simulink library "EngineSystemSubmodel"  (Simulink 8.1)
settings: Solver=ode45  StartTime=0.0  StopTime=10.0  FixedStep=1e-4  RelTol=1e-3
values from neighbouring files (symbols this model uses):
  B = [B1;B2]    [GensetRespOptimiztion.m]    (also in GensetRespOptimiztionTorstein.m; Init8RTFLEX68D.m = 0.68; init_MVM.m = 0.127)
  beta = 0.75    [Init8RTFLEX68D.m]
  cAStartRef = 104.8    [Init8RTFLEX68D.m]
  coeffMechEff = [0.135;0.155]    [Init8RTFLEX68D.m]
  comp_eff_map = [0 0 0 0 0 0 0 0 0 0 0 0 ... (250000 elements, 500x500)]    [comp_map.mat]    (also in comp_mapABB A175-35L.mat)
  comp_flow_map = [0 0 0 0 0 0 0 0 0 0 0 0 ... (250000 elements, 500x500)]    [comp_map.mat]    (also in comp_mapABB A175-35L.mat)
  D_turb_wheel = TC.TC_map.turb.D_wheel    [init_MVM.m]
  dCALiftDown = cAVVDownRef(end) - cAVVDownRef(1)    [Init8RTFLEX68D.m]
  dCALiftTopRef = 63.5    [Init8RTFLEX68D.m]
  dCALiftUp = cAVVUpRef(end) - cAVVUpRef(1)    [Init8RTFLEX68D.m]
  Dp = 0.383    [Init8RTFLEX68D.m]
  Ds = 0.079    [Init8RTFLEX68D.m]
  Dv = 0.425    [Init8RTFLEX68D.m]
  eff_coeff = [-1.0889528323728;0.91854258409396;-0.10659748546926;                     0.21229452390244;-0.053186221596493;-0.005451194709834]    [Init8RTFLEX68D.m]
  eta_turb_max = TC.TC_map.turb.eff_max    [init_MVM.m]
  flow_coeff_turb = [-1.585326540339;-4.823836967181;1.5853156139822]    [Init8RTFLEX68D.m]    (also in init_MVM.m = TC.TC_map.turb.flow_fit_coeff)
  fs = 0.0683    [Init8RTFLEX68D.m]    (also in NOxProcessGUI.m = varargin{2}; initHybrid.m; initMV.m; init_MVM.m = 0.0682925799315)
  genset = generators(1)    [runTempCyl4S.m]
  J_tc = TC.SAE_map_comp.inertia    [init_MVM.m]
  jShaft = 0    [EngineSystemParameters.m]    (also in Init8RTFLEX68D.m = 323000)
  jTC = 2    [Init8RTFLEX68D.m]
  Kb = 1*ones(engines,1)    [initHybrid.m]    (also in initMV.m; init_MVM.m = 1; init_ele.m = 1)
  Kd = 20*ones(engines,1)    [initHybrid.m]    (also in initMV.m; init_MVM.m = 10; init_ele.m = 20)
  Ki = 20*ones(engines,1)    [initHybrid.m]    (also in initMV.m; init_MVM.m = 10; init_ele.m = 20)
  Kp = 20*ones(engines,1)    [initHybrid.m]    (also in initMV.m; init_MVM.m = 10; init_ele.m = 20)
  lambdaCrank = 0.5056    [Init8RTFLEX68D.m]
  liftMax = 0.17    [Init8RTFLEX68D.m]
  Load_amp = x(4) + xRef(i)    [GetErrGensetResp.m]    (also in runsimulation.m = 0.55; runsimulationRecovery.m = InitialLoad(jj) + LoadStep(ii))
  Load_bias = x(4)    [GetErrGensetResp.m]    (also in runsimulation.m = 0.15; runsimulationRecovery.m = InitialLoad(jj))
  Load_index = 1    [GetErrGensetResp.m]    (also in runsimulation.m; runsimulationRecovery.m)
  mqfCycMax = 9.5547e-2    (= 0.095547)    [Init8RTFLEX68D.m]
  N = x*noMol    [NOxProcessGUI.m]    (also in initHybrid.m = .1*ones(engines,1); initMV.m = .1*ones(engines,1); init_ele.m = 0.1)
  n288_rep = [0 222.054 444.108 666.162 888.216 1110.27 1332.324 1554.378 1776.432 1998.486 2220.54 2442.594 ... (500 elements, 1x500)]    [comp_map.mat]
  nPort = 28    [Init8RTFLEX68D.m]
  npr = length(pr_rep)    [Init8RTFLEX68D.m]    (also in initHybrid.m; initMV.m; init_MVM.m)
  nsp = length(n288_rep)    [Init8RTFLEX68D.m]    (also in initHybrid.m; initMV.m; init_MVM.m)
  nStroke = 2    [Init8RTFLEX68D.m]
  omegat0 = RPM_TC_initial/30*pi    [init_MVM.m]
  pr_rep = [1.01 1.0150249672 1.0200499344 1.0250749016 1.0300998688 1.035124836 1.0401498032 1.0451747704 1.0501997376 1.0552247048 1.060249672 1.0652746392 ... (500 elements, 1x500)]    [comp_map.mat]
  r = 0.035    [Init8RTFLEX68D.m]
  Start_time = 50    [GetErrGensetResp.m]    (also in runsimulation.m; runsimulationRecovery.m)
  stroke = 2.72    [Init8RTFLEX68D.m]
  T_load = 1    [GetErrGensetResp.m]    (also in runsimulation.m; runsimulationRecovery.m)
  T_ref_turb = TC.TC_map.turb.T_ref    [init_MVM.m]
  u0 = 0.2    [init_MVM.m]
  Uc_opt = TC.TC_map.turb.Uc_opt    [init_MVM.m]
  w = 0.021    [Init8RTFLEX68D.m]
  wasteGateMax = 10    [Init8RTFLEX68D.m]
  wasteGateMin = 0    [Init8RTFLEX68D.m]
  wiebePara = [0.07;0.57;3.05;11;24;56.3;1.5;1;0.7]    [Init8RTFLEX68D.m]
  X = 0.07    [Init8RTFLEX68D.m]
  Y = 0.16    [Init8RTFLEX68D.m]
undefined symbols (not defined in the file or in its folder): aCrank, cAVVDownRef, cAVVUpRef, liftDownRef, liftUpRef, omega0, Td, Ti, u_max
undefined symbols (not defined in the file): BWdmExhBypass, cAlpha, cCylHT, E0A, ECyl0, hn, KbWG, KpWG, lowerCloseSPWG, m0A, mb0A, mbCyl0, mCp, mCyl0, nCyl, phi0, phi0A, phi0rad, RPM0, RPMMax, RPMT0, TiWG, upperOpenWG, V0A, vCyl0, wasteGateRatio
libraries: EngineSystemSubmodel x49, simulink x1
(part 1 of 3)
settings Model: Creator=yum  LastModifiedBy=yum

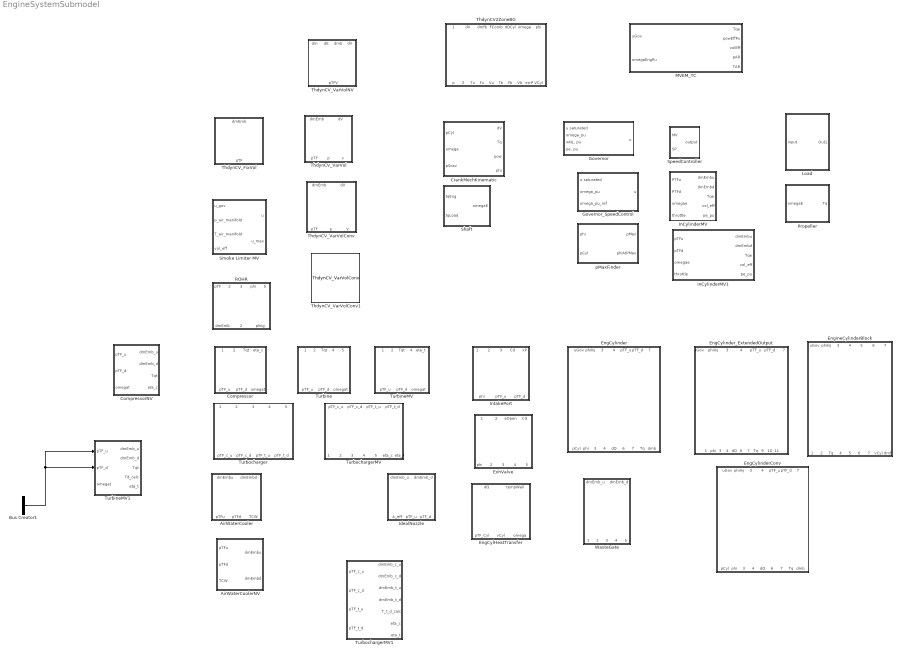
== system EngineSystemSubmodel ==
  AirWaterCooler : Subsystem  mask{fs=0, Cd=0, A_air_path=0, dm_cw=0, coeff_T_cw_K=0, Cp_cw=0, D_cw_pipe=0}
      mask prompts: fs "Stoichiometric fuel-air ratio"; Cd "Discharge coefficient (0.8)"; A_air_path "Effective sectional area of air path (m2)"; dm_cw "Coolant flow rate (kg/s)"; coeff_T_cw_K "Coefficient for effective heat transfer area w.r.t. coolant temperature (2x1)"; Cp_cw "Specific heat capacity of coolant"; D_cw_pipe "Pipe diameter of the cooling water pipe in the cooler (m)"
      mask TypeOptions fs: S-Function/fs
      mask TypeOptions Cd: S-Function/Cd
      mask TypeOptions A_air_path: S-Function/A_air_path
      mask TypeOptions dm_cw: S-Function/dm_cw
      mask TypeOptions coeff_T_cw_K: S-Function/coeff_T_cw_K
      mask TypeOptions Cp_cw: S-Function/Cp_cw
      mask TypeOptions D_cw_pipe: S-Function/D_cw_pipe
  AirWaterCoolerNV : Subsystem  mask{fs=0, Cd=0, A_air_path=0, dm_cw=0, coeff_T_cw_K=0, Cp_cw=0, D_cw_pipe=0}
      mask prompts: fs "Stoichiometric fuel-air ratio"; Cd "Discharge coefficient (0.8)"; A_air_path "Effective sectional area of air path (m2)"; dm_cw "Coolant flow rate (kg/s)"; coeff_T_cw_K "Coefficient for effective heat transfer area w.r.t. coolant temperature (2x1)"; Cp_cw "Specific heat capacity of coolant"; D_cw_pipe "Pipe diameter of the cooling water pipe in the cooler (m)"
      mask TypeOptions fs: S-Function/fs
      mask TypeOptions Cd: S-Function/Cd
      mask TypeOptions A_air_path: S-Function/A_air_path
      mask TypeOptions dm_cw: S-Function/dm_cw
      mask TypeOptions coeff_T_cw_K: S-Function/coeff_T_cw_K
      mask TypeOptions Cp_cw: S-Function/Cp_cw
      mask TypeOptions D_cw_pipe: S-Function/D_cw_pipe
  Bus Creator1 : BusCreator  Inputs=3
  Compressor : Subsystem  mask{fs=0, comp_flow_map=0, comp_eff_map=0, pr_rep=0, n288_rep=0, npr=0, nsp=0}
      mask prompts: fs "Fuel-air equivalent ratio"; comp_flow_map "Compressor map for corrected flow"; comp_eff_map "Compressor map for efficiency"; pr_rep "Pressure ratio array for look-up in compressor map"; n288_rep "Corrected speed array for look-up in compressor map"; npr "Length of pressure ratio array for look-up in compressor map"; nsp "Length of corrected speed array for look-up in compressor map"
  CompressorNV : Subsystem  mask{fs=0, comp_flow_map=0, comp_eff_map=0, pr_rep=0, n288_rep=0, npr=0, nsp=0}
      mask prompts: fs "Fuel-air equivalent ratio"; comp_flow_map "Compressor map for corrected flow"; comp_eff_map "Compressor map for efficiency"; pr_rep "Pressure ratio array for look-up in compressor map"; n288_rep "Corrected speed array for look-up in compressor map"; npr "Length of pressure ratio array for look-up in compressor map"; nsp "Length of corrected speed array for look-up in compressor map"
  CrankMechKinematic : Subsystem  mask{phi0=0, B=0, stroke=0, lambdaCrank=0}
      mask prompts: phi0 "Initial crank angle"; B "Bore of the cylinder"; lambdaCrank "Ratio of length of crank rod to that of connecting rod"
      mask TypeOptions phi0: S-Function/phi0
      mask TypeOptions B: S-Function/B
      mask TypeOptions stroke: S-Function/stroke
      mask TypeOptions lambdaCrank: S-Function/lambdaCrank
  EngCylHeatTransfer : Subsystem  mask{stroke=0, B=0, cAlpha=0, mCp=0, cCylHT=0, nCyl=0, tempWall0=0}
      mask prompts: stroke "Storke [m]"; B "Bore [m]"; cAlpha "Fitting coefficient for convective heat transfer coefficient"; mCp "Heat capacity of the cylinder [J/K]"; cCylHT "Polynomial coefficient for heat rejection model from the cylinder (4 x 1)"; nCyl "Number of cylinders"; tempWall0 "Initial cylinder wall temperature"
      mask TypeOptions stroke: S-Function/stroke
      mask TypeOptions B: S-Function/B
      mask TypeOptions cAlpha: S-Function/cAlpha
      mask TypeOptions mCp: S-Function/mCp
      mask TypeOptions cCylHT: S-Function/cCylHT
      mask TypeOptions nCyl: S-Function/nCyl
      mask TypeOptions tempWall0: S-Function/tempWall0
  EngCylinder : Subsystem  mask{fs=fs, nStroke=nStroke, hn=hn, nCyl=nCyl, iCyl=2, B=B, stroke=stroke, lambdaCrank=lambdaCrank, aCrank=aCrank, X=X, Y=Y, r=r, nPort=nPort, liftMax=liftMax, Dv=Dv, beta=beta, w=w, Dp=Dp, Ds=Ds, cAVVUpRef=cAVVUpRef, cAVVDownRef=cAVVDownRef, liftUpRef=liftUpRef, liftDownRef=liftDownRef, cAStartRef=cAStartRef, dCALiftUp=dCALiftUp, dCALiftDown=dCALiftDown, dCALiftTopRef=dCALiftTopRef, mCp=mCp, cCylHT=cCylHT, cAlpha=cAlpha, mqfCycMax=mqfCycMax, wiebePara=wiebePara, phi0=phi0, m0=mCyl0, E0=ECyl0, mb0=mbCyl0, V0=vCyl0, phi0A=phi0A, m0A=m0A, E0A=E0A, mb0A=mb0A, V0A=V0A}
      mask prompts: fs "Stoichiometric fuel-air ratio"; nStroke "Number of stroke"; hn "Lower heating value of the fuel [J/kg]"; nCyl "Number of cylinders"; iCyl "Cylinder number"; B "Bore of the cylinder [m]"; stroke "Stroke [m]"; lambdaCrank "Ratio of length of crank rod to connecting rod"; aCrank "Length of crank rod [m]"; X "Width of inport opening [m]"; Y "Height of inport opening [m]"; r "Raidus of fillet of the opening"; nPort "Number of ports [pcs]"; liftMax "Maximum valve lift [m]"; Dv "Valve head diameter [m]"; beta "Seat angle [rad]"; w "Valve seat width [m]"; Dp "Inner seat diameter [m]"; Ds "Stem diameter [m]"; cAVVUpRef "Crank angle array for opening [deg]"; cAVVDownRef "Crank angle array for closing [deg]"; liftUpRef "Normalized lift array for opening (0~1)"; liftDownRef "Normalized lift array for closing (0~1)"; cAStartRef "Nominal crank angle at start of valve lif [deg]"; dCALiftUp "Nominal duration of crank angle for valve opening [deg]"; dCALiftDown "Nominal duration of crank angle for valve closing [deg]"; dCALiftTopRef "Nominal duration of crank angle for valve open [deg]"; mCp "Heat capacity of the cylinder [J/K]"; cCylHT "Polynomial coefficient for heat rejection model from the cylinder (4 x 1)"; cAlpha "Fitting coefficient for convective heat transfer coefficient"; mqfCycMax "Maximum fuel mass injected per cycle [kg]"; wiebePara "3-Wiebe Parameters (9x1)"; phi0 "Initial crank angle [deg]"; m0 "Initial mass [kg]"; E0 "Initial internal energy [J]"; mb0 "Initial burned fuel mass [kg]"; V0 "Initial volume [m3]"; phi0A "Initial crank angle array [deg]"; m0A "Initial mass array [kg]"; E0A "Initial internal energy array [J]"; mb0A "Initial burned fuel mass array [kg]"; V0A "Initial volume array [m3]"
      mask init:
      | CylNo = uint8(iCyl);
      | if CylNo > 0 
      |     phi0 = phi0A(CylNo);
      |     m0 = m0A(CylNo);
      |     E0 = E0A(CylNo);
      |     mb0 = mb0A(CylNo);
      |     V0 = V0A(CylNo);
      | else
      |     phi0 = phi0A(1);
      |     m0 = m0A(1);
      |     E0 = E0A(1);
      |     mb0 = mb0A(1);
      |     V0 = V0A(1);
      | end;
      mask TypeOptions fs: ThdynCV_VarVol1/fs | IntakePort1/fs | ExhValve/fs
      mask TypeOptions nStroke: IntakePort1/nStroke
      mask TypeOptions hn: ROHR1/hn
      mask TypeOptions nCyl: EngCylHeatTransfer/nCyl
      mask TypeOptions B: CrankMechKinematic/B | EngCylHeatTransfer/B
      mask TypeOptions stroke: CrankMechKinematic/stroke | EngCylHeatTransfer/stroke | IntakePort1/stroke
      mask TypeOptions lambdaCrank: IntakePort1/lambdaCrank | CrankMechKinematic/lambdaCrank
      mask TypeOptions aCrank: IntakePort1/aCrank
      mask TypeOptions X: IntakePort1/X
      mask TypeOptions Y: IntakePort1/Y
      mask TypeOptions r: IntakePort1/r
      mask TypeOptions nPort: IntakePort1/nPort
      mask TypeOptions liftMax: ExhValve/liftMax
      mask TypeOptions Dv: ExhValve/Dv
      mask TypeOptions beta: ExhValve/beta
      mask TypeOptions w: ExhValve/w
      mask TypeOptions Dp: ExhValve/Dp
      mask TypeOptions Ds: ExhValve/Ds
      mask TypeOptions cAVVUpRef: ExhValve/cAVVUpRef
      mask TypeOptions cAVVDownRef: ExhValve/cAVVDownRef
      mask TypeOptions liftUpRef: ExhValve/liftUpRef
      mask TypeOptions liftDownRef: ExhValve/liftDownRef
      mask TypeOptions cAStartRef: ExhValve/cAStartRef
      mask TypeOptions dCALiftUp: ExhValve/dCALiftUp
      mask TypeOptions dCALiftDown: ExhValve/dCALiftDown
      mask TypeOptions dCALiftTopRef: ExhValve/dCALiftTopRef
      mask TypeOptions mCp: EngCylHeatTransfer/mCp
      mask TypeOptions cCylHT: EngCylHeatTransfer/cCylHT
      mask TypeOptions cAlpha: EngCylHeatTransfer/cAlpha
      mask TypeOptions mqfCycMax: ROHR1/mqfCycMax
      mask TypeOptions wiebePara: ROHR1/wiebePara
      mask TypeOptions phi0: CrankMechKinematic/phi0
      mask TypeOptions m0: ThdynCV_VarVol1/m0
      mask TypeOptions E0: ThdynCV_VarVol1/E0
      mask TypeOptions mb0: ThdynCV_VarVol1/mb0
      mask TypeOptions V0: ThdynCV_VarVol1/V0
  EngCylinderConv : Subsystem  mask{fs=fs, nStroke=2, hn=hn, nCyl=nCyl, iCyl=2, B=B, stroke=stroke, lambdaCrank=lambdaCrank, aCrank=stroke/2, X=X, Y=Y, r=r, nPort=nPort, liftMax=liftMax, Dv=Dv, beta=beta, w=w, Dp=Dp, Ds=Ds, cAVVUpRef=cAVVUpRef, cAVVDownRef=cAVVDownRef, liftUpRef=liftUpRef, liftDownRef=liftDownRef, cAStartRef=cAStartRef, dCALiftUp=dCALiftUp, dCALiftDown=dCALiftDown, dCALiftTopRef=dCALiftTopRef, mCp=mCp, cCylHT=cCylHT, cAlpha=cAlpha, mqfCycMax=mqfCycMax, wiebePara=wiebePara, phi0=phi0, p0=0, T0=0, F0=0, V0=0, phi0A=phi0A, p0A=m0A, T0A=E0A, F0A=mb0A, V0A=V0A}
      mask prompts: fs "Stoichiometric fuel-air ratio"; nStroke "Number of stroke"; hn "Lower heating value of the fuel [J/kg]"; nCyl "Number of cylinders"; iCyl "Cylinder number"; B "Bore of the cylinder [m]"; stroke "Stroke [m]"; lambdaCrank "Ratio of length of crank rod to connecting rod"; aCrank "Length of crank rod [m]"; X "Width of inport opening [m]"; Y "Height of inport opening [m]"; r "Raidus of fillet of the opening"; nPort "Number of ports [pcs]"; liftMax "Maximum valve lift [m]"; Dv "Valve head diameter [m]"; beta "Seat angle [rad]"; w "Valve seat width [m]"; Dp "Inner seat diameter [m]"; Ds "Stem diameter [m]"; cAVVUpRef "Crank angle array for opening [deg]"; cAVVDownRef "Crank angle array for closing [deg]"; liftUpRef "Normalized lift array for opening (0~1)"; liftDownRef "Normalized lift array for closing (0~1)"; cAStartRef "Nominal crank angle at start of valve lif [deg]"; dCALiftUp "Nominal duration of crank angle for valve opening [deg]"; dCALiftDown "Nominal duration of crank angle for valve closing [deg]"; dCALiftTopRef "Nominal duration of crank angle for valve open [deg]"; mCp "Heat capacity of the cylinder [J/K]"; cCylHT "Polynomial coefficient for heat rejection model from the cylinder (4 x 1)"; cAlpha "Fitting coefficient for convective heat transfer coefficient"; mqfCycMax "Maximum fuel mass injected per cycle [kg]"; wiebePara "3-Wiebe Parameters (9x1)"; phi0 "Initial crank angle [deg]"; p0 "Initial pressure [Pa]"; T0 "Initial temperature [K]"; F0 "Initial fuel-air equivalent ratio"; V0 "Initial volume [m3]"; phi0A "Initial crank angle array [deg]"; p0A "Initial pressure array [Pa]"; T0A "Initial temperature array [J]"; F0A "Initial fuel-air equivalent ratio array"; V0A "Initial volume array [m3]"
      mask init:
      | CylNo = uint8(iCyl);
      | if CylNo > 0 
      |     phi0 = phi0A(CylNo);
      |     p0 = p0A(CylNo);
      |     T0 = T0A(CylNo);
      |     F0 = F0A(CylNo);
      |     V0 = V0A(CylNo);
      | else
      |     phi0 = phi0A(1);
      |     p0 = p0A(1);
      |     T0 = T0A(1);
      |     F0 = F0A(1);
      |     V0 = V0A(1);
      | end;
      mask TypeOptions fs: ExhValve/fs | IntakePort1/fs | ThdynCV_VarVolConv/fs
      mask TypeOptions nStroke: IntakePort1/nStroke
      mask TypeOptions hn: ROHR1/hn
      mask TypeOptions nCyl: EngCylHeatTransfer/nCyl
      mask TypeOptions B: CrankMechKinematic/B | EngCylHeatTransfer/B
      mask TypeOptions stroke: CrankMechKinematic/stroke | EngCylHeatTransfer/stroke | IntakePort1/stroke
      mask TypeOptions lambdaCrank: IntakePort1/lambdaCrank | CrankMechKinematic/lambdaCrank
      mask TypeOptions aCrank: IntakePort1/aCrank
      mask TypeOptions X: IntakePort1/X
      mask TypeOptions Y: IntakePort1/Y
      mask TypeOptions r: IntakePort1/r
      mask TypeOptions nPort: IntakePort1/nPort
      mask TypeOptions liftMax: ExhValve/liftMax
      mask TypeOptions Dv: ExhValve/Dv
      mask TypeOptions beta: ExhValve/beta
      mask TypeOptions w: ExhValve/w
      mask TypeOptions Dp: ExhValve/Dp
      mask TypeOptions Ds: ExhValve/Ds
      mask TypeOptions cAVVUpRef: ExhValve/cAVVUpRef
      mask TypeOptions cAVVDownRef: ExhValve/cAVVDownRef
      mask TypeOptions liftUpRef: ExhValve/liftUpRef
      mask TypeOptions liftDownRef: ExhValve/liftDownRef
      mask TypeOptions cAStartRef: ExhValve/cAStartRef
      mask TypeOptions dCALiftUp: ExhValve/dCALiftUp
      mask TypeOptions dCALiftDown: ExhValve/dCALiftDown
      mask TypeOptions dCALiftTopRef: ExhValve/dCALiftTopRef
      mask TypeOptions mCp: EngCylHeatTransfer/mCp
      mask TypeOptions cCylHT: EngCylHeatTransfer/cCylHT
      mask TypeOptions cAlpha: EngCylHeatTransfer/cAlpha
      mask TypeOptions mqfCycMax: ROHR1/mqfCycMax
      mask TypeOptions wiebePara: ROHR1/wiebePara
      mask TypeOptions phi0: CrankMechKinematic/phi0
      mask TypeOptions p0: ThdynCV_VarVolConv/p0
      mask TypeOptions T0: ThdynCV_VarVolConv/T0
      mask TypeOptions F0: ThdynCV_VarVolConv/F0
      mask TypeOptions V0: ThdynCV_VarVolConv/V0
  EngCylinder_ExtendedOutput : Subsystem  mask{fs=fs, nStroke=nStroke, hn=hn, nCyl=nCyl, iCyl=1, B=B, stroke=stroke, lambdaCrank=lambdaCrank, aCrank=aCrank, X=X, Y=Y, r=r, nPort=nPort, liftMax=liftMax, Dv=Dv, beta=beta, w=w, Dp=Dp, Ds=Ds, cAVVUpRef=cAVVUpRef, cAVVDownRef=cAVVDownRef, liftUpRef=liftUpRef, liftDownRef=liftDownRef, cAStartRef=cAStartRef, dCALiftUp=dCALiftUp, dCALiftDown=dCALiftDown, dCALiftTopRef=dCALiftTopRef, mCp=mCp, cCylHT=cCylHT, cAlpha=cAlpha, mqfCycMax=mqfCycMax, wiebePara=wiebePara, phi0=phi0, m0=mCyl0, E0=ECyl0, mb0=mbCyl0, V0=vCyl0, phi0A=phi0A, m0A=m0A, E0A=E0A, mb0A=mb0A, V0A=V0A}
      mask prompts: fs "Stoichiometric fuel-air ratio"; nStroke "Number of stroke"; hn "Lower heating value of the fuel [J/kg]"; nCyl "Number of cylinders"; iCyl "Cylinder number"; B "Bore of the cylinder [m]"; stroke "Stroke [m]"; lambdaCrank "Ratio of length of crank rod to connecting rod"; aCrank "Length of crank rod [m]"; X "Width of inport opening [m]"; Y "Height of inport opening [m]"; r "Raidus of fillet of the opening"; nPort "Number of ports [pcs]"; liftMax "Maximum valve lift [m]"; Dv "Valve head diameter [m]"; beta "Seat angle [rad]"; w "Valve seat width [m]"; Dp "Inner seat diameter [m]"; Ds "Stem diameter [m]"; cAVVUpRef "Crank angle array for opening [deg]"; cAVVDownRef "Crank angle array for closing [deg]"; liftUpRef "Normalized lift array for opening (0~1)"; liftDownRef "Normalized lift array for closing (0~1)"; cAStartRef "Nominal crank angle at start of valve lif [deg]"; dCALiftUp "Nominal duration of crank angle for valve opening [deg]"; dCALiftDown "Nominal duration of crank angle for valve closing [deg]"; dCALiftTopRef "Nominal duration of crank angle for valve open [deg]"; mCp "Heat capacity of the cylinder [J/K]"; cCylHT "Polynomial coefficient for heat rejection model from the cylinder (4 x 1)"; cAlpha "Fitting coefficient for convective heat transfer coefficient"; mqfCycMax "Maximum fuel mass injected per cycle [kg]"; wiebePara "3-Wiebe Parameters (9x1)"; phi0 "Initial crank angle [deg]"; m0 "Initial mass [kg]"; E0 "Initial internal energy [J]"; mb0 "Initial burned fuel mass [kg]"; V0 "Initial volume [m3]"; phi0A "Initial crank angle array [deg]"; m0A "Initial mass array [kg]"; E0A "Initial internal energy array [J]"; mb0A "Initial burned fuel mass array [kg]"; V0A "Initial volume array [m3]"
      mask init: same as EngineSystemSubmodel/EngCylinder
      mask TypeOptions fs: ThdynCV_VarVol1/fs | IntakePort1/fs | ExhValve/fs
      mask TypeOptions nStroke: IntakePort1/nStroke
      mask TypeOptions hn: ROHR1/hn
      mask TypeOptions nCyl: EngCylHeatTransfer/nCyl
      mask TypeOptions B: CrankMechKinematic/B | EngCylHeatTransfer/B
      mask TypeOptions stroke: CrankMechKinematic/stroke | EngCylHeatTransfer/stroke | IntakePort1/stroke
      mask TypeOptions lambdaCrank: IntakePort1/lambdaCrank | CrankMechKinematic/lambdaCrank
      mask TypeOptions aCrank: IntakePort1/aCrank
      mask TypeOptions X: IntakePort1/X
      mask TypeOptions Y: IntakePort1/Y
      mask TypeOptions r: IntakePort1/r
      mask TypeOptions nPort: IntakePort1/nPort
      mask TypeOptions liftMax: ExhValve/liftMax
      mask TypeOptions Dv: ExhValve/Dv
      mask TypeOptions beta: ExhValve/beta
      mask TypeOptions w: ExhValve/w
      mask TypeOptions Dp: ExhValve/Dp
      mask TypeOptions Ds: ExhValve/Ds
      mask TypeOptions cAVVUpRef: ExhValve/cAVVUpRef
      mask TypeOptions cAVVDownRef: ExhValve/cAVVDownRef
      mask TypeOptions liftUpRef: ExhValve/liftUpRef
      mask TypeOptions liftDownRef: ExhValve/liftDownRef
      mask TypeOptions cAStartRef: ExhValve/cAStartRef
      mask TypeOptions dCALiftUp: ExhValve/dCALiftUp
      mask TypeOptions dCALiftDown: ExhValve/dCALiftDown
      mask TypeOptions dCALiftTopRef: ExhValve/dCALiftTopRef
      mask TypeOptions mCp: EngCylHeatTransfer/mCp
      mask TypeOptions cCylHT: EngCylHeatTransfer/cCylHT
      mask TypeOptions cAlpha: EngCylHeatTransfer/cAlpha
      mask TypeOptions mqfCycMax: ROHR1/mqfCycMax
      mask TypeOptions wiebePara: ROHR1/wiebePara
      mask TypeOptions phi0: CrankMechKinematic/phi0
      mask TypeOptions m0: ThdynCV_VarVol1/m0
      mask TypeOptions E0: ThdynCV_VarVol1/E0
      mask TypeOptions mb0: ThdynCV_VarVol1/mb0
      mask TypeOptions V0: ThdynCV_VarVol1/V0
  EngineCylinderBlock : Subsystem  mask{fs=fs, nStroke=nStroke, hn=hn, nCyl=nCyl, B=B, stroke=stroke, lambdaCrank=lambdaCrank, aCrank=stroke/2, X=X, Y=Y, r=r, nPort=nPort, liftMax=liftMax, Dv=Dv, beta=beta, w=w, Dp=Dp, Ds=Ds, cAVVUpRef=cAVVUpRef, cAVVDownRef=cAVVDownRef, liftUpRef=liftUpRef, liftDownRef=liftDownRef, cAStartRef=cAStartRef, dCALiftUp=dCALiftUp, dCALiftDown=dCALiftDown, dCALiftTopRef=dCALiftTopRef, mCp=mCp, cCylHT=cCylHT, cAlpha=cAlpha, mqfCycMax=mqfCycMax, wiebePara=wiebePara, phi0A=phi0rad, m0A=mCyl0, E0A=ECyl0, mb0A=mbCyl0, V0A=vCyl0}
      mask prompts: fs "Stoichiometric fuel-air ratio"; nStroke "Number of stroke"; hn "Lower heating value of the fuel [J/kg]"; nCyl "Number of cylinders"; B "Bore of the cylinder [m]"; stroke "Stroke [m]"; lambdaCrank "Ratio of length of crank rod to connecting rod"; aCrank "Length of crank rod [m]"; X "Width of inport opening [m]"; Y "Height of inport opening [m]"; r "Raidus of fillet of the opening"; nPort "Number of ports [pcs]"; liftMax "Maximum valve lift [m]"; Dv "Valve head diameter [m]"; beta "Seat angle [rad]"; w "Valve seat width [m]"; Dp "Inner seat diameter [m]"; Ds "Stem diameter [m]"; cAVVUpRef "Crank angle array for opening [deg]"; cAVVDownRef "Crank angle array for closing [deg]"; liftUpRef "Normalized lift array for opening (0~1)"; liftDownRef "Normalized lift array for closing (0~1)"; cAStartRef "Nominal crank angle at start of valve lif [deg]"; dCALiftUp "Nominal duration of crank angle for valve opening [deg]"; dCALiftDown "Nominal duration of crank angle for valve closing [deg]"; dCALiftTopRef "Nominal duration of crank angle for valve open [deg]"; mCp "Heat capacity of the cylinder [J/K]"; cCylHT "Polynomial coefficient for heat rejection model from the cylinder (4 x 1)"; cAlpha "Fitting coefficient for convective heat transfer coefficient"; mqfCycMax "Maximum fuel mass injected per cycle [kg]"; wiebePara "3-Wiebe Parameters (9x1)"; phi0A "Initial crank angle array [deg]"; m0A "Initial mass array [kg]"; E0A "Initial internal energy array [J]"; mb0A "Initial burned fuel mass array [kg]"; V0A "Initial volume array [m3]"
      mask TypeOptions fs: EngCylinder1/fs | EngCylinder2/fs | EngCylinder3/fs | EngCylinder4/fs | EngCylinder5/fs | EngCylinder6/fs | EngCylinder7/fs | EngCylinder8/fs
      mask TypeOptions nStroke: EngCylinder1/nStroke | EngCylinder2/nStroke | EngCylinder3/nStroke | EngCylinder4/nStroke | EngCylinder5/nStroke | EngCylinder6/nStroke | EngCylinder7/nStroke | EngCylinder8/nStroke
      mask TypeOptions hn: EngCylinder1/hn | EngCylinder2/hn | EngCylinder3/hn | EngCylinder4/hn | EngCylinder5/hn | EngCylinder6/hn | EngCylinder7/hn | EngCylinder8/hn
      mask TypeOptions nCyl: EngCylinder1/nCyl | EngCylinder2/nCyl | EngCylinder3/nCyl | EngCylinder4/nCyl | EngCylinder5/nCyl | EngCylinder6/nCyl | EngCylinder7/nCyl | EngCylinder8/nCyl
      mask TypeOptions B: EngCylinder1/B | EngCylinder2/B | EngCylinder3/B | EngCylinder4/B | EngCylinder5/B | EngCylinder6/B | EngCylinder7/B | EngCylinder8/B
      mask TypeOptions stroke: EngCylinder1/stroke | EngCylinder2/stroke | EngCylinder3/stroke | EngCylinder4/stroke | EngCylinder5/stroke | EngCylinder6/stroke | EngCylinder7/stroke | EngCylinder8/stroke
      mask TypeOptions lambdaCrank: EngCylinder1/lambdaCrank | EngCylinder2/lambdaCrank | EngCylinder3/lambdaCrank | EngCylinder4/lambdaCrank | EngCylinder5/lambdaCrank | EngCylinder6/lambdaCrank | EngCylinder7/lambdaCrank | EngCylinder8/lambdaCrank
      mask TypeOptions aCrank: EngCylinder1/aCrank | EngCylinder2/aCrank | EngCylinder3/aCrank | EngCylinder4/aCrank | EngCylinder5/aCrank | EngCylinder6/aCrank | EngCylinder7/aCrank | EngCylinder8/aCrank
      mask TypeOptions X: EngCylinder1/X | EngCylinder2/X | EngCylinder3/X | EngCylinder4/X | EngCylinder5/X | EngCylinder6/X | EngCylinder7/X | EngCylinder8/X
      mask TypeOptions Y: EngCylinder1/Y | EngCylinder2/Y | EngCylinder3/Y | EngCylinder4/Y | EngCylinder5/Y | EngCylinder6/Y | EngCylinder7/Y | EngCylinder8/Y
      mask TypeOptions r: EngCylinder1/r | EngCylinder2/r | EngCylinder3/r | EngCylinder4/r | EngCylinder5/r | EngCylinder6/r | EngCylinder7/r | EngCylinder8/r
      mask TypeOptions nPort: EngCylinder1/nPort | EngCylinder2/nPort | EngCylinder3/nPort | EngCylinder4/nPort | EngCylinder5/nPort | EngCylinder6/nPort | EngCylinder7/nPort | EngCylinder8/nPort
      mask TypeOptions liftMax: EngCylinder1/liftMax | EngCylinder2/liftMax | EngCylinder3/liftMax | EngCylinder4/liftMax | EngCylinder5/liftMax | EngCylinder6/liftMax | EngCylinder7/liftMax | EngCylinder8/liftMax
      mask TypeOptions Dv: EngCylinder2/Dv | EngCylinder3/Dv | EngCylinder1/Dv | EngCylinder4/Dv | EngCylinder5/Dv | EngCylinder6/Dv | EngCylinder7/Dv | EngCylinder8/Dv
      mask TypeOptions beta: EngCylinder1/beta | EngCylinder2/beta | EngCylinder3/beta | EngCylinder4/beta | EngCylinder5/beta | EngCylinder6/beta | EngCylinder7/beta | EngCylinder8/beta
      mask TypeOptions w: EngCylinder1/w | EngCylinder2/w | EngCylinder3/w | EngCylinder4/w | EngCylinder5/w | EngCylinder6/w | EngCylinder7/w | EngCylinder8/w
      mask TypeOptions Dp: EngCylinder1/Dp | EngCylinder2/Dp | EngCylinder3/Dp | EngCylinder4/Dp | EngCylinder5/Dp | EngCylinder6/Dp | EngCylinder7/Dp | EngCylinder8/Dp
      mask TypeOptions Ds: EngCylinder1/Ds | EngCylinder2/Ds | EngCylinder3/Ds | EngCylinder4/Ds | EngCylinder5/Ds | EngCylinder6/Ds | EngCylinder7/Ds | EngCylinder8/Ds
      mask TypeOptions cAVVUpRef: EngCylinder1/cAVVUpRef | EngCylinder2/cAVVUpRef | EngCylinder3/cAVVUpRef | EngCylinder4/cAVVUpRef | EngCylinder5/cAVVUpRef | EngCylinder6/cAVVUpRef | EngCylinder7/cAVVUpRef | EngCylinder8/cAVVUpRef
      mask TypeOptions cAVVDownRef: EngCylinder1/cAVVDownRef | EngCylinder2/cAVVDownRef | EngCylinder3/cAVVDownRef | EngCylinder4/cAVVDownRef | EngCylinder5/cAVVDownRef | EngCylinder6/cAVVDownRef | EngCylinder7/cAVVDownRef | EngCylinder8/cAVVDownRef
      mask TypeOptions liftUpRef: EngCylinder1/liftUpRef | EngCylinder2/liftUpRef | EngCylinder3/liftUpRef | EngCylinder4/liftUpRef | EngCylinder5/liftUpRef | EngCylinder6/liftUpRef | EngCylinder7/liftUpRef | EngCylinder8/liftUpRef
      mask TypeOptions liftDownRef: EngCylinder1/liftDownRef | EngCylinder2/liftDownRef | EngCylinder3/liftDownRef | EngCylinder4/liftDownRef | EngCylinder5/liftDownRef | EngCylinder6/liftDownRef | EngCylinder7/liftDownRef | EngCylinder8/liftDownRef
      mask TypeOptions cAStartRef: EngCylinder1/cAStartRef | EngCylinder2/cAStartRef | EngCylinder3/cAStartRef | EngCylinder4/cAStartRef | EngCylinder5/cAStartRef | EngCylinder6/cAStartRef | EngCylinder7/cAStartRef | EngCylinder8/cAStartRef
      mask TypeOptions dCALiftUp: EngCylinder1/dCALiftUp | EngCylinder2/dCALiftUp | EngCylinder3/dCALiftUp | EngCylinder4/dCALiftUp | EngCylinder5/dCALiftUp | EngCylinder6/dCALiftUp | EngCylinder7/dCALiftUp | EngCylinder8/dCALiftUp
      mask TypeOptions dCALiftDown: EngCylinder1/dCALiftDown | EngCylinder2/dCALiftDown | EngCylinder3/dCALiftDown | EngCylinder4/dCALiftDown | EngCylinder5/dCALiftDown | EngCylinder6/dCALiftDown | EngCylinder7/dCALiftDown | EngCylinder8/dCALiftDown
      mask TypeOptions dCALiftTopRef: EngCylinder1/dCALiftTopRef | EngCylinder2/dCALiftTopRef | EngCylinder3/dCALiftTopRef | EngCylinder4/dCALiftTopRef | EngCylinder5/dCALiftTopRef | EngCylinder6/dCALiftTopRef | EngCylinder7/dCALiftTopRef | EngCylinder8/dCALiftTopRef
      mask TypeOptions mCp: EngCylinder1/mCp | EngCylinder2/mCp | EngCylinder3/mCp | EngCylinder4/mCp | EngCylinder5/mCp | EngCylinder6/mCp | EngCylinder7/mCp | EngCylinder8/mCp
      mask TypeOptions cCylHT: EngCylinder1/cCylHT | EngCylinder2/cCylHT | EngCylinder3/cCylHT | EngCylinder4/cCylHT | EngCylinder5/cCylHT | EngCylinder6/cCylHT | EngCylinder7/cCylHT | EngCylinder8/cCylHT
      mask TypeOptions cAlpha: EngCylinder1/cAlpha | EngCylinder2/cAlpha | EngCylinder3/cAlpha | EngCylinder4/cAlpha | EngCylinder5/cAlpha | EngCylinder6/cAlpha | EngCylinder7/cAlpha | EngCylinder8/cAlpha
      mask TypeOptions mqfCycMax: EngCylinder1/mqfCycMax | EngCylinder2/mqfCycMax | EngCylinder3/mqfCycMax | EngCylinder4/mqfCycMax | EngCylinder5/mqfCycMax | EngCylinder6/mqfCycMax | EngCylinder7/mqfCycMax | EngCylinder8/mqfCycMax
      mask TypeOptions wiebePara: EngCylinder1/wiebePara | EngCylinder2/wiebePara | EngCylinder3/wiebePara | EngCylinder4/wiebePara | EngCylinder5/wiebePara | EngCylinder6/wiebePara | EngCylinder7/wiebePara | EngCylinder8/wiebePara
      mask TypeOptions phi0A: EngCylinder1/phi0A | EngCylinder2/phi0A | EngCylinder3/phi0A | EngCylinder4/phi0A | EngCylinder5/phi0A | EngCylinder6/phi0A | EngCylinder7/phi0A | EngCylinder8/phi0A
      mask TypeOptions m0A: EngCylinder1/m0A | EngCylinder2/m0A | EngCylinder3/m0A | EngCylinder4/m0A | EngCylinder5/m0A | EngCylinder6/m0A | EngCylinder7/m0A | EngCylinder8/m0A
      mask TypeOptions E0A: EngCylinder1/E0A | EngCylinder2/E0A | EngCylinder3/E0A | EngCylinder4/E0A | EngCylinder5/E0A | EngCylinder6/E0A | EngCylinder7/E0A | EngCylinder8/E0A
      mask TypeOptions mb0A: EngCylinder1/mb0A | EngCylinder2/mb0A | EngCylinder3/mb0A | EngCylinder4/mb0A | EngCylinder5/mb0A | EngCylinder6/mb0A | EngCylinder7/mb0A | EngCylinder8/mb0A
      mask TypeOptions V0A: EngCylinder1/V0A | EngCylinder2/V0A | EngCylinder3/V0A | EngCylinder4/V0A | EngCylinder5/V0A | EngCylinder6/V0A | EngCylinder7/V0A | EngCylinder8/V0A
  ExhValve : Subsystem  mask{fs=0, cAVVUpRef=0, cAVVDownRef=0, liftUpRef=0, liftDownRef=0, cAStartRef=0, dCALiftUp=0, dCALiftDown=0, dCALiftTopRef=0, liftMax=0, Dv=0, beta=0, w=0, Dp=0, Ds=0}
      mask prompts: fs "Stoichiometric fuel-air equivalent ratio"; cAVVUpRef "Crank angle array for opening [deg]"; cAVVDownRef "Crank angle array for closing [deg]"; liftUpRef "Normalized lift array for opening (0~1)"; liftDownRef "Normalized lift array for closing (0~1)"; cAStartRef "Nominal crank angle at start of valve lif [deg]"; dCALiftUp "Nominal duration of crank angle for valve opening [deg]"; dCALiftDown "Nominal duration of crank angle for valve closing [deg]"; dCALiftTopRef "Nominal duration of crank angle for valve open [deg]"; liftMax "Maximum valve lift [m]"; Dv "Valve head diameter [m]"; beta "Seat angle [rad]"; w "Valve seat width [m]"; Dp "Inner seat diameter [m]"; Ds "Stem diameter [m]"
      mask TypeOptions fs: IdealNozzle/fs
      mask TypeOptions cAVVUpRef: S-Function/cAVVUpRef
      mask TypeOptions cAVVDownRef: S-Function/cAVVDownRef
      mask TypeOptions liftUpRef: S-Function/liftUpRef
      mask TypeOptions liftDownRef: S-Function/liftDownRef
      mask TypeOptions cAStartRef: S-Function/cAStartRef
      mask TypeOptions dCALiftUp: S-Function/dCALiftUp
      mask TypeOptions dCALiftDown: S-Function/dCALiftDown
      mask TypeOptions dCALiftTopRef: S-Function/dCALiftTopRef
      mask TypeOptions liftMax: S-Function/liftMax
      mask TypeOptions Dv: S-Function1/Dv
      mask TypeOptions beta: S-Function1/beta
      mask TypeOptions w: S-Function1/w
      mask TypeOptions Dp: S-Function1/Dp
      mask TypeOptions Ds: S-Function1/Ds
  Governor : Subsystem
  Governor_SpeedControl : Subsystem  mask{Kp=Kp, Kd=Kd, N=0, Ki=Ki, Kb=Kb, omega0=omega0, u_min=u_max, u_max=u_max, u0=u0}
      mask prompts: Kp "Proportional gain"; Kd "Differential gain"; N "Dirty derivative gain"; Ki "Integral gain"; Kb "Back-calculation gain"; omega0 "Initial engine speed [pu]"; u_min "Minimum governor output"; u_max "Maximum governor output"; u0 "Initial governor output"
      mask TypeOptions Kp: PID controller/Kp
      mask TypeOptions Kd: PID controller/Kd
      mask TypeOptions N: PID controller/N
      mask TypeOptions Ki: PID controller/Ki
      mask TypeOptions Kb: PID controller/Kb
      mask TypeOptions omega0: PID controller/omega0
      mask TypeOptions u_min: PID controller/u_min
      mask TypeOptions u_max: PID controller/u_max
      mask TypeOptions u0: PID controller/u0
  IdealNozzle : Subsystem  mask{fs=[]}
      mask prompts: fs "Stoichiometric fuel-air equivalent ratio"
  InCylinderMV : Subsystem  mask{fs=0, Vd=0, LHV=0, Pe_nom=0, SFC=0, vol_eff_coeff1=0, vol_eff_coeff2=0, T_pe=0, nstroke=0, m_f_cyc_max=0, C1=0, p_a_inf=0, Pe0=0}
      mask prompts: fs "Stoichiometric fuel-air ratio"; Vd "Displacement volume (m3)"; LHV "Lower heating value of the fuel (J/kg)"; Pe_nom "Rated shaft power (W)"; SFC "Quadratic SFC curve coefficient (3x1)"; vol_eff_coeff1 "Volumetric efficiency coefficient for higher inlet pressure"; vol_eff_coeff2 "Volumetric efficiency coefficient for lower inlet pressure"; T_pe "Time constant for the torque development"; nstroke "Number of stroke"; m_f_cyc_max "Maximum amount of fuel injected per cycle (kg)"; C1 "Heat loss coefficient"; p_a_inf "Upper pressure limit for volumetric efficiency model 1 [bar]"; Pe0 "Initial power"
      mask TypeOptions fs: S-Function/fs
      mask TypeOptions Vd: S-Function/Vd
      mask TypeOptions LHV: S-Function/LHV
      mask TypeOptions Pe_nom: S-Function/Pe_nom
      mask TypeOptions SFC: S-Function/SFC
      mask TypeOptions vol_eff_coeff1: S-Function/vol_eff_coeff1
      mask TypeOptions vol_eff_coeff2: S-Function/vol_eff_coeff2
      mask TypeOptions T_pe: S-Function/T_pe
      mask TypeOptions nstroke: S-Function/nstroke
      mask TypeOptions m_f_cyc_max: S-Function/m_f_cyc_max
      mask TypeOptions C1: S-Function/C1
      mask TypeOptions p_a_inf: S-Function/p_a_inf
      mask TypeOptions Pe0: S-Function/Pe0
  InCylinderMV1 : Subsystem  mask{fs=genset.eng.fs, Vd=genset.eng.vD, LHV=genset.eng.LHV, Pe_nom=genset.eng.powNom, SFC=genset.eng.SFC, vol_eff_coeff1=genset.eng.volEff1, vol_eff_coeff2=genset.eng.volEff2, T_pe=genset.eng.tPe, nstroke=genset.eng.nStroke, m_f_cyc_max=genset.eng.mFCycMax, C1=genset.eng.C1, p_a_inf=genset.eng.pAInf, Pe0=genset.eng.powL0*genset.eng.powNom}
      mask prompts: fs "Stoichiometric fuel-air ratio"; Vd "Displacement volume (m3)"; LHV "Lower heating value of the fuel (J/kg)"; Pe_nom "Rated shaft power (W)"; SFC "Quadratic SFC curve coefficient (3x1)"; vol_eff_coeff1 "Volumetric efficiency coefficient for higher inlet pressure"; vol_eff_coeff2 "Volumetric efficiency coefficient for lower inlet pressure"; T_pe "Time constant for the torque development"; nstroke "Number of stroke"; m_f_cyc_max "Maximum amount of fuel injected per cycle (kg)"; C1 "Heat loss coefficient"; p_a_inf "Upper pressure limit for volumetric efficiency model 1 [bar]"; Pe0 "Initial power"
      mask TypeOptions fs: S-Function/fs
      mask TypeOptions Vd: S-Function/Vd
      mask TypeOptions LHV: S-Function/LHV
      mask TypeOptions Pe_nom: S-Function/Pe_nom
      mask TypeOptions SFC: S-Function/SFC
      mask TypeOptions vol_eff_coeff1: S-Function/vol_eff_coeff1
      mask TypeOptions vol_eff_coeff2: S-Function/vol_eff_coeff2
      mask TypeOptions T_pe: S-Function/T_pe
      mask TypeOptions nstroke: S-Function/nstroke
      mask TypeOptions m_f_cyc_max: S-Function/m_f_cyc_max
      mask TypeOptions C1: S-Function/C1
      mask TypeOptions p_a_inf: S-Function/p_a_inf
      mask TypeOptions Pe0: S-Function/Pe0
  IntakePort : Subsystem  mask{fs=0, nStroke=0, aCrank=0, lambdaCrank=0, X=0, Y=0, r=0, nPort=0, stroke=0}
      mask prompts: fs "Stoichiometric fuel-air equivalent ratio"; nStroke "Number of stroke"; aCrank "Length of crank rod [m]"; lambdaCrank "Ratio of length of a crank rod to connecting rod"; X "Width of inport opening [m]"; Y "Height of inport opening [m]"; r "Raidus of fillet of the opening"; nPort "Number of ports [pcs]"; stroke "Stroke [m]"
      mask TypeOptions fs: IdealNozzle/fs
      mask TypeOptions nStroke: S-Function/nStroke
      mask TypeOptions aCrank: S-Function/aCrank
      mask TypeOptions lambdaCrank: S-Function/lambdaCrank
      mask TypeOptions X: S-Function/X
      mask TypeOptions Y: S-Function/Y
      mask TypeOptions r: S-Function/r
      mask TypeOptions nPort: S-Function/nPort
      mask TypeOptions stroke: S-Function/stroke
  Load : Subsystem  mask{Load_index=Load_index, Load_amp=Load_amp, Load_bias=Load_bias, Start_time=Start_time, T_load=T_load}
      mask prompts: Load_index "Load index"; Load_amp "Load amplitude"; Load_bias "Load in bias"; Start_time "Load initiation time"; T_load "Period of the load"
      mask help:
      | Load Selection and Definition
      | Load_index   Load_amp   Load_bias   Start_time    T_load
      | 1-Step,             Final,      Initial,        Step time,      N/A,
      | 2-Sine,             amp,        bias,           Delay,          Period
      | 3-Ramp,             Slope,      Initial,        Start time,     N/A
      | 4-User input        N/A,        Initial,        Delay,          N/A
      | 5-External input    N/A,        Initial,        Delay,          N/A
      | 6-Constant          N/A,        Load,           N/A,            N/A
  MVEM_TC : Subsystem  mask{genset=genset}
      mask prompts: genset "Genset parameters"
  Propeller : MATLAB Function  TreatAsAtomicUnit=on
  ROHR : Subsystem  mask{mqfCycMax=mqfCycMax, wiebePara=wiebePara, hn=hn}
      mask prompts: mqfCycMax "Maximum fuel mass injected per cycle [kg]"; wiebePara "3-Wiebe Parameters"; hn "Lower heating value of the fuel [J/kg]"
      mask TypeOptions mqfCycMax: S-Function/mqfCycMax
      mask TypeOptions wiebePara: S-Function/wiebePara | S-Function1/wiebePara
      mask TypeOptions hn: S-Function1/hn
  Shaft : Subsystem  mask{jShaft=jShaft, HShaft=0, omegaEMax=RPMMax*pi/30, coeffMechEff=coeffMechEff, omegaE0=RPM0*pi/30}
      mask prompts: jShaft "Mass moment of inertia of the shaft [kgm2]"; HShaft "Inverse of mass moment of inertia of the shaft (1/J) [kg-1m-2]"; omegaEMax "Maximum engine speed (rad/s)"; coeffMechEff "Coefficient for mechanical efficiency model (2x1)"; omegaE0 "Initial engine speed [rad/s]"
      mask init:
      | HShaft = 1/jShaft;
      mask TypeOptions jShaft: Integrator/jShaft
      mask TypeOptions HShaft: Gain/HShaft
      mask TypeOptions omegaEMax: MATLAB Function/omegaEMax
      mask TypeOptions coeffMechEff: MATLAB Function/coeffMechEff
      mask TypeOptions omegaE0: Integrator/omegaE0
  Smoke Limiter MV : Subsystem  mask{fs=genset.eng.fs, Vd=genset.eng.vD, F_max=genset.eng.fMax, m_f_cyc_max=genset.eng.mFCycMax}
      mask prompts: fs "Stoichiometric fuel-air ratio"; Vd "Displacement volume (m3)"; F_max "Maximum fuel-air equivalent ratio"; m_f_cyc_max "Maximum fuel injection @ rated power (kg)"
  SpeedController : Subsystem  mask(20-sim 4.4 S-Function block){}
      mask help:
      | This block is generated by the 20-sim ANSI-C Code Generator.
      |
      | * look under the mask to get information on the ports
      | * press Help for more detailed information
      | * the parameters of this block are:
      mask Help:
      | This block is generated by the 20-sim ANSI-C Code Generator<br>
      | The block parameters are:<br><blockquote></blockquote>
      | Generated at:<br>
      | <blockquote><b>date:  </b>August 27, 2014<br>
      | <b>time:  </b>10:21:01 pm<br></blockquote>
      | From the following 20-sim model:<br>
      | <blockquote><b>submodel:  </b>SpeedController<br>
      | <b>model:  </b>8RT-FLEX68-D_transient<br>
      | <b>file:  </b>E:\DBox\Dropbox\Study\Research Project\SHI Project\Program\BG\8RT-FLEX68-D_transient.emx<br>
      | <b>experiment:  </b>E:\DBox\Dropbox\Study\Research Project\SHI Project\Program\BG\8RT-FLEX68-D_transient.emx<br></blockquote>
      | Using the following 20-sim license:<br>
      | <blockquote><b>user:  </b>Norwegian University of Science and Technology <br>
      | <b>from:  </b>20-sim 4.4 Student License<br>
      | <b>build: </b>4.4.1.4356<br></blockquote>
      mask Display:
      | patch ([928 992 992 928 928 ], [184 184 248 248 184 ], [0.901965 0.901965 0.901965] )
      | color ('black ')
      | plot ([928 992 992 928 928 ], [184 184 248 248 184 ])
      | color ('blue')
      | text (972.3,217,'PID','hor','center')
      | color ('blue')
      | text (940.8,233.1,'SP','hor','center')
      | color ('blue')
      | text (942.9,202.1,'MV','hor','center')
      | color ('black')
      | text (985.6,195.7,'p','hor','center')
  ThdynCV2ZoneBG : Subsystem  mask{fs=0, DPhiMix=0, phiMix0=0, alpha=0, hn=0, p0=0, T0=0, F0=0, V0=0}
      mask prompts: fs "Stoichiometric fuel-air ratio"; DPhiMix "Duration of mixing from burned zone to unburned zone [deg]"; phiMix0 "Start of mixing from burned zone to unburend [deg]"; alpha "Ratio of burned mass to unburned during gas exchange"; hn "Low heating value of the fuel [J/kg]"; p0 "Initial pressure [Pa]"; T0 "Initial temperature [K]"; F0 "Initial fuel-air equivalent ratio"; V0 "Initial volume [m3]"
      mask TypeOptions fs: S-Function/fs
      mask TypeOptions DPhiMix: S-Function/DPhiMix
      mask TypeOptions phiMix0: S-Function/phiMix0
      mask TypeOptions alpha: S-Function/alpha
      mask TypeOptions hn: S-Function/hn
      mask TypeOptions p0: S-Function/p0
      mask TypeOptions T0: S-Function/T0
      mask TypeOptions F0: S-Function/F0
      mask TypeOptions V0: S-Function/V0
  ThdynCV_FixVol : Subsystem  mask{fs=0, m0=0, E0=0, mb0=0, V=0}
      mask prompts: fs "Stoichiometric fuel-air ratio"; m0 "Initial mass (kg)"; E0 "Initial internal energy (J)"; mb0 "Initial burned fuel mass (kg)"; V "Volume (m3)"
  ThdynCV_VarVol : Subsystem  mask{fs=0, m0=0, E0=0, mb0=0, V0=0}
      mask prompts: fs "Stoichiometric fuel-air ratio"; m0 "Initial mass (kg)"; E0 "Initial internal energy (J)"; mb0 "Initial burned fuel mass (kg)"; V0 "Initial volume (m3)"
  ThdynCV_VarVolConv : Subsystem  mask{fs=0, p0=0, T0=0, F0=0, V0=0}
      mask prompts: fs "Stoichiometric fuel-air ratio"; p0 "Initial pressure"; T0 "Initial temperature"; F0 "Initial fuel-air equivalent ratio"; V0 "Initial volume"
      mask TypeOptions fs: S-Function/fs
      mask TypeOptions p0: S-Function/p0
      mask TypeOptions T0: S-Function/T0
      mask TypeOptions F0: S-Function/F0
      mask TypeOptions V0: S-Function/V0
  ThdynCV_VarVolConv1 : EngineSystemSubmodel/ThdynCV_VarVolConv  fs=0  p0=0  T0=0  F0=0  V0=0
  ThdynCV_VarVolNV : Subsystem  mask{fs=0, m0=0, E0=0, mb0=0, V0=0}
      mask prompts: fs "Stoichiometric fuel-air ratio"; m0 "Initial mass (kg)"; E0 "Initial internal energy (J)"; mb0 "Initial burned fuel mass (kg)"; V0 "Initial volume (m3)"
  Turbine : Subsystem  mask{fs=0, flow_coeff_turb=0, eff_coeff=0}
      mask prompts: fs "Fuel-Air equivalent ratio"; flow_coeff_turb "Turbine flow coefficient"; eff_coeff "Turbine efficient coefficient"
      mask TypeOptions fs: S-Function/fs
      mask TypeOptions flow_coeff_turb: S-Function/flow_coeff_turb
      mask TypeOptions eff_coeff: S-Function/eff_coeff
  TurbineMV : Subsystem  mask{fs=0, flow_coeff_turb=0, D_turb_wheel=0, Uc_opt=0, eta_turb_max=0}
      mask prompts: fs "Stoichiometric fuel-air ratio"; flow_coeff_turb "Flow coefficient for turbine model (3x1)"; D_turb_wheel "Turbine wheel diameter (m)"; Uc_opt "Optimal blade speed ratio"; eta_turb_max "Maximum efficiency"
  TurbineMV1 : Subsystem  mask{fs=0, flow_coeff_turb=0, D_turb_wheel=0, Uc_opt=0, eta_turb_max=0, T_ref_turb=0}
      mask prompts: fs "Stoichiometric fuel-air ratio"; flow_coeff_turb "Flow coefficient for turbine model (3x1)"; D_turb_wheel "Turbine wheel diameter (m)"; Uc_opt "Optimal blade speed ratio"; eta_turb_max "Maximum efficiency"; T_ref_turb "Reference temperature"
  Turbocharger : Subsystem  mask{fs=fs, jTC=jTC, comp_flow_map=comp_flow_map, comp_eff_map=comp_eff_map, pr_rep=pr_rep, n288_rep=n288_rep, npr=npr, nsp=nsp, flow_coeff_turb=flow_coeff_turb, eff_coeff=eff_coeff, omegat0=RPMT0 * pi / 30}
      mask prompts: fs "Stoichiometric fuel-air ratio"; jTC "Mass moment of inertia of a rotor (kgm2)"; comp_flow_map "Compressor map for corrected flow"; comp_eff_map "Compressor map for efficiency"; pr_rep "Pressure ratio array for look-up in compressor map"; n288_rep "Corrected speed array for look-up in compressor map"; npr "Length of pressure ratio array for look-up in compressor map"; nsp "Length of corrected speed array for look-up in compressor map"; flow_coeff_turb "Turbine flow coefficient"; eff_coeff "Turbine efficient coefficient"; omegat0 "Initial rotating speed (rad/s)"
      mask TypeOptions fs: Compressor1/fs | Turbine1/fs
      mask TypeOptions comp_flow_map: Compressor1/comp_flow_map
      mask TypeOptions comp_eff_map: Compressor1/comp_eff_map
      mask TypeOptions pr_rep: Compressor1/pr_rep
      mask TypeOptions n288_rep: Compressor1/n288_rep
      mask TypeOptions npr: Compressor1/npr
      mask TypeOptions nsp: Compressor1/nsp
      mask TypeOptions flow_coeff_turb: Turbine1/flow_coeff_turb
      mask TypeOptions eff_coeff: Turbine1/eff_coeff
  TurbochargerMV : Subsystem  mask{fs=fs, J_tc=J_tc, omegat0=omegat0, comp_flow_map=comp_flow_map, comp_eff_map=comp_eff_map, pr_rep=pr_rep, n_288_rep=n288_rep, npr=npr, nsp=nsp, flow_coeff_turb=flow_coeff_turb, D_wheel_turb=D_turb_wheel, Uc_opt=Uc_opt, eta_turb_max=eta_turb_max, T_ref=T_ref_turb}
      mask prompts: fs "Stoichiometric fuel-air ratio"; J_tc "Mass moment of inertia of a rotor"; omegat0 "Initial rotor speed"; comp_flow_map "Compressor map for corrected flow"; comp_eff_map "Compressor map for efficiency"; pr_rep "Pressure ratio arry for look-up in compressor map"; n_288_rep "Corrected speed array for look-up in compressor map"; npr "Length of pressure ratio array for look-up in compressor map"; nsp "Length of corrected speed array for look-up in compressor map"; flow_coeff_turb "Flow coefficient for turbine model"; D_wheel_turb "Turbine wheel diameter"; Uc_opt "Optimal blade speed ratio"; eta_turb_max "Maximum efficiency"; T_ref "Reference temperature for turbine flow"
  TurbochargerMV1 : Subsystem  AncestorBlock=EngineSystemSubmodel/TurbochargerMV  mask{fs=fs, J_tc=J_tc, omegat0=omegat0, comp_flow_map=comp_flow_map, comp_eff_map=comp_eff_map, pr_rep=pr_rep, n_288_rep=n288_rep, npr=npr, nsp=nsp, flow_coeff_turb=flow_coeff_turb, D_wheel_turb=D_turb_wheel, Uc_opt=Uc_opt, eta_turb_max=eta_turb_max, T_ref=T_ref_turb}
      mask prompts: fs "Stoichiometric fuel-air ratio"; J_tc "Mass moment of inertia of a rotor"; omegat0 "Initial rotor speed"; comp_flow_map "Compressor map for corrected flow"; comp_eff_map "Compressor map for efficiency"; pr_rep "Pressure ratio arry for look-up in compressor map"; n_288_rep "Corrected speed array for look-up in compressor map"; npr "Length of pressure ratio array for look-up in compressor map"; nsp "Length of corrected speed array for look-up in compressor map"; flow_coeff_turb "Flow coefficient for turbine model"; D_wheel_turb "Turbine wheel diameter"; Uc_opt "Optimal blade speed ratio"; eta_turb_max "Maximum efficiency"; T_ref "Reference temperature for turbine flow"
  WasteGate : Subsystem  mask{fs=fs, Kp=KpWG, Ti=TiWG, K_b=KbWG, max=wasteGateMax, min=wasteGateMin, bypassRatio=wasteGateRatio, upper=upperOpenWG, lower=lowerCloseSPWG, BWdmExhBypass=BWdmExhBypass, BWdmExh=BWdmExhBypass}
      mask prompts: fs "Stoichiometric fuel-air equivalent ratio"; Kp "Proportional gain"; Ti "Integral time constant"; K_b "Back calculation gain for anti-windup"; max "Maximum allowable valve opening"; min "Maximum allowable valve opening"; bypassRatio "Bypass ratio"; upper "Upper bound for opening waste gate"; lower "Lower bound for closing waste gate"; BWdmExhBypass "The bandwidth of the LP filter for bypass flow [Hz]"; BWdmExh "The bandwidth of the LP filter for exhaust flow [Hz]"
      mask TypeOptions fs: IdealNozzle/fs
      mask TypeOptions Kp: wasteGateControl/Kp
      mask TypeOptions Ti: wasteGateControl/Ti
      mask TypeOptions K_b: wasteGateControl/K_b
      mask TypeOptions max: wasteGateControl/max
      mask TypeOptions min: wasteGateControl/min
      mask TypeOptions bypassRatio: wasteGateControl/bypassRatio
      mask TypeOptions upper: wasteGateControl/upper
      mask TypeOptions lower: wasteGateControl/lower
      mask TypeOptions BWdmExhBypass: S-Function/BW
      mask TypeOptions BWdmExh: S-Function1/BW
  pMaxFinder : Subsystem
  wires:
  Bus Creator1/1 -> TurbineMV1/2(pTF_d), TurbineMV1/1(pTF_u)
  ? -> Bus Creator1/1  "p"
  ? -> Bus Creator1/2  "T"
  ? -> Bus Creator1/3  "F"
